simulink model "final_quadruped_120722"  (R2021a)
settings: Solver=ode15s  StartTime=0.0  StopTime=10  FixedStep=1e-3  RelTol=1e-5  EnableMultiTasking=on
values from neighbouring files (symbols this model uses):
  foot_x = 8    [bipedparameters.m]    (also in fcn.m; finalrobotParameters.m; finalrobotParameters_110522.m; finalrobotParameters_140522.m)
  foot_y = 6    [bipedparameters.m]    (also in fcn.m; finalrobotParameters.m; finalrobotParameters_110522.m; finalrobotParameters_140522.m)
  foot_z = 1    [bipedparameters.m]    (also in fcn.m; finalrobotParameters.m; finalrobotParameters_110522.m; finalrobotParameters_140522.m)
  height_plane = 0.025    [bipedparameters.m]    (also in finalrobotParameters.m; finalrobotParameters_110522.m; finalrobotParameters_140522.m; finalrobotParameters_240522.m)
  kd_ankle = 1000    [bipedparameters.m]    (also in finalrobotParameters_240522.m)
  kd_hip = 1000    [bipedparameters.m]    (also in finalrobotParameters_240522.m)
  kd_knee = 1000    [bipedparameters.m]    (also in finalrobotParameters_240522.m)
  ki_ankle = 1000    [bipedparameters.m]    (also in finalrobotParameters_240522.m)
  ki_hip = 1000    [bipedparameters.m]    (also in finalrobotParameters_240522.m)
  ki_knee = 2000    [bipedparameters.m]    (also in finalrobotParameters_240522.m)
  kp_ankle = 1000    [bipedparameters.m]    (also in finalrobotParameters_240522.m)
  kp_hip = 1000    [bipedparameters.m]    (also in finalrobotParameters_240522.m)
  kp_knee = 2000    [bipedparameters.m]    (also in finalrobotParameters_240522.m)
  lower_leg_length = 10    [bipedparameters.m]    (also in fcn.m; finalrobotParameters.m; finalrobotParameters_110522.m; finalrobotParameters_140522.m)
  plane_x = 25    [bipedparameters.m]    (also in finalrobotParameters.m; finalrobotParameters_110522.m; finalrobotParameters_140522.m; finalrobotParameters_240522.m)
  plane_y = 3    [bipedparameters.m]    (also in finalrobotParameters.m; finalrobotParameters_110522.m; finalrobotParameters_140522.m; finalrobotParameters_240522.m)
  torso_offset_x = -0.5    [bipedparameters.m]    (also in finalrobotParameters.m = 10; finalrobotParameters_110522.m = 10; finalrobotParameters_140522.m = 10; finalrobotParameters_240522.m = 10)
  torso_offset_z = -2    [bipedparameters.m]    (also in finalrobotParameters.m; finalrobotParameters_110522.m; finalrobotParameters_140522.m; finalrobotParameters_240522.m)
  torso_x = 5    [bipedparameters.m]    (also in fcn.m = 25; finalrobotParameters.m = 25; finalrobotParameters_110522.m = 25; finalrobotParameters_140522.m = 25)
  torso_y = 10    [bipedparameters.m]    (also in fcn.m = 16; finalrobotParameters.m = 16; finalrobotParameters_110522.m = 16; finalrobotParameters_140522.m = 16)
  torso_z = 8    [bipedparameters.m]    (also in fcn.m = 10; finalrobotParameters.m = 10; finalrobotParameters_110522.m = 10; finalrobotParameters_140522.m = 10)
  upper_leg_length = 10    [bipedparameters.m]    (also in fcn.m; finalrobotParameters.m; finalrobotParameters_110522.m; finalrobotParameters_140522.m)
undefined symbols (not defined in the file or in its folder): sigbuilder_block, X, Y, Z
libraries: nesl_utility x288, sm_lib x75, pid_lib x20, Contact_Forces_Lib x16, fl_lib x3
(part 2 of 9)

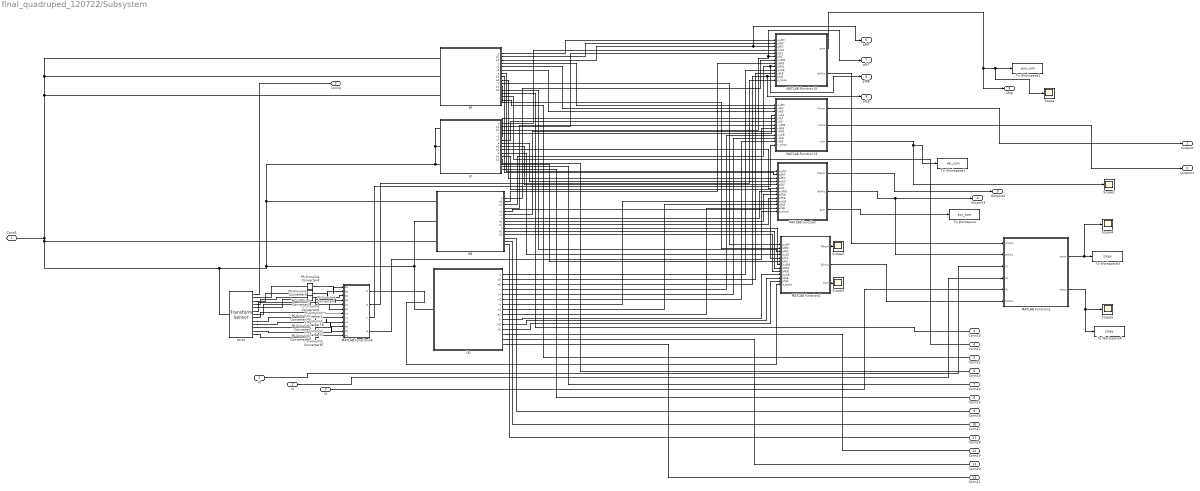
== system final_quadruped_120722/Subsystem ==
  I3 : Inport
  I4 : Inport  Port=2
  I5 : Inport  Port=3
  " RF" : Subsystem
  LB : Subsystem
  LF : Subsystem
  MATLAB Function : MATLAB Function  TreatAsAtomicUnit=on
  MATLAB Function1 : MATLAB Function  TreatAsAtomicUnit=on
  MATLAB Function13 : MATLAB Function  TreatAsAtomicUnit=on
  MATLAB Function14 : MATLAB Function  TreatAsAtomicUnit=on
  MATLAB Function15 : MATLAB Function  TreatAsAtomicUnit=on
  MATLAB Function2 : MATLAB Function  TreatAsAtomicUnit=on
  PS-Simulink Converter{,1..6,76..78,86..87} (12 alike) : nesl_utility/PS-Simulink Converter  PhysicalDomain=network_engine_domain  SubClassName=ps_output  LeftPortType=input  RightPortType=output  PseudoPeriodic=off  Frequencies=[]  Unit=inherit  AffineConversion=off
      settings: SourceProductBaseCode=PW,SS
  RB : Subsystem
  Scope{,1..5} (6 alike) : Scope
  To Workspace : ToWorkspace  VariableName=acc_com  SaveFormat=Timeseries  SampleTime=-1
  To Workspace1 : ToWorkspace  VariableName=vel_com  SaveFormat=Timeseries  SampleTime=-1
  To Workspace2 : ToWorkspace  VariableName=pos_com  SaveFormat=Timeseries  SampleTime=-1
  To Workspace3 : ToWorkspace  VariableName=zmpx  SaveFormat=Timeseries  SampleTime=-1
  To Workspace4 : ToWorkspace  VariableName=zmpy  SaveFormat=Timeseries  SampleTime=-1
  torso : sm_lib/Frames and Transforms/Transform Sensor  MeasurementFrame=World  SenseAngle=off  SenseAxis=off  SenseAngle1=off  SenseAngle2=off  SenseAngle3=off  SenseQ=off  SenseR=off  SenseOmegaX=off  SenseOmegaY=off  SenseOmegaZ=off  SenseOmega1=off  SenseOmega2=off  SenseOmega3=off  SenseQDot=off  SenseRDot=off  SenseAlphaX=on  SenseAlphaY=on  SenseAlphaZ=on  SenseAlpha1=off  SenseAlpha2=off  SenseAlpha3=off  SenseQDDot=off  SenseRDDot=off  SenseX=on  SenseY=on  SenseZ=on  SenseRad=off  SenseAzim=off  SenseDist=off  SenseInc=off  SenseXDot=on  SenseYDot=on  SenseZDot=on  SenseRadDot=off  SenseAzimDot=off  SenseDistDot=off  SenseIncDot=off  SenseXDDot=on  SenseYDDot=on  SenseZDDot=on  SenseRadDDot=off  SenseAzimDDot=off  SenseDistDDot=off  SenseIncDDot=off
  Conn5 : PMIOPort  Side=Left
  Conn4 : PMIOPort  Port=2  Side=Right
  Conn10 : PMIOPort  Port=3  Side=Right
  Conn11 : PMIOPort  Port=4  Side=Right
  Conn12 : PMIOPort  Port=5  Side=Right
  Conn13 : PMIOPort  Port=6  Side=Right
  Conn14 : PMIOPort  Port=7  Side=Right
  Conn15 : PMIOPort  Port=8  Side=Right
  Conn16 : PMIOPort  Port=9  Side=Right
  Conn17 : PMIOPort  Port=10  Side=Right
  Conn18 : PMIOPort  Port=11  Side=Right
  Conn19 : PMIOPort  Port=12  Side=Right
  Conn20 : PMIOPort  Port=13  Side=Right
  Conn21 : PMIOPort  Port=14  Side=Right
  Outport : Outport
  Outport1 : Outport  Port=2
  Outport2 : Outport  Port=3
  Outport3 : Outport  Port=4
  CMg : Outport  Port=5
  pfRF : Outport  Port=6
  pfLF : Outport  Port=7
  pfRB : Outport  Port=8
  pfLB : Outport  Port=9
  wires:
  PS-Simulink Converter3/1 -> MATLAB Function14/4(px)
  PS-Simulink Converter1/1 -> MATLAB Function14/5(py)
  PS-Simulink Converter2/1 -> MATLAB Function14/6(pz)
  MATLAB Function14/3(v) -> MATLAB Function13/13(v_torso)
  MATLAB Function13/1(Mvcm) -> Outport/1
  MATLAB Function13/2(vlinks) -> Outport1/1
  PS-Simulink Converter78/1 -> MATLAB Function14/7(vx)
  PS-Simulink Converter76/1 -> MATLAB Function14/8(vy)
  PS-Simulink Converter77/1 -> MATLAB Function14/9(vz)
  MATLAB Function14/4(a) -> MATLAB Function/13(a_torso)
  MATLAB Function/1(Macm) -> Outport2/1
  MATLAB Function/2(alinks) -> MATLAB Function1/2(alinks), Outport3/1
  MATLAB Function/3(acm) -> To Workspace/1
  MATLAB Function13/3(vcm) -> Scope1/1, To Workspace1/1
  PS-Simulink Converter/1 -> MATLAB Function14/10(ax)
  PS-Simulink Converter87/1 -> MATLAB Function14/11(ay)
  PS-Simulink Converter86/1 -> MATLAB Function14/12(az)
  MATLAB Function14/2(p) -> MATLAB Function15/13(p_torso)
  MATLAB Function15/1(pcm) -> CMg/1, Scope/1, To Workspace2/1
  " RF"/1(p) -> MATLAB Function15/1(pulRF)
  " RF"/2(p1) -> MATLAB Function15/2(pllRF)
  " RF"/3(p2) -> pfRF/1, MATLAB Function15/3(pfRF)
  " RF"/4(v) -> MATLAB Function13/1(vulRF)
  " RF"/5(v1) -> MATLAB Function13/2(vllRF)
  " RF"/6(v2) -> MATLAB Function13/3(vfRF)
  " RF"/7(a) -> MATLAB Function/1(aulRF)
  " RF"/8(a1) -> MATLAB Function/2(allRF)
  " RF"/9(a2) -> MATLAB Function/3(afRF)
  RB/1(p) -> MATLAB Function15/7(pulRB)
  RB/2(p1) -> MATLAB Function15/8(pllRB)
  RB/3(p2) -> pfRB/1, MATLAB Function15/9(pfRB)
  RB/4(v) -> MATLAB Function13/7(vulRB)
  RB/5(v1) -> MATLAB Function13/8(vllRB)
  RB/6(v2) -> MATLAB Function13/9(vfRB)
  RB/7(a) -> MATLAB Function/7(aulRB)
  RB/8(a1) -> MATLAB Function/8(allRB)
  RB/9(a2) -> MATLAB Function/9(afRB)
  LF/1(p) -> MATLAB Function15/4(pulLF)
  LF/2(p1) -> MATLAB Function15/5(pllLF)
  LF/3(p2) -> pfLF/1, MATLAB Function15/6(pfLF)
  LF/4(v) -> MATLAB Function13/4(vulLF)
  LF/5(v1) -> MATLAB Function13/5(vllLF)
  LF/6(v2) -> MATLAB Function13/6(vfLF)
  LF/7(a) -> MATLAB Function/4(aulLF)
  LF/8(a1) -> MATLAB Function/5(allLF)
  LF/9(a2) -> MATLAB Function/6(afLF)
  LB/1(p) -> MATLAB Function15/10(pulLB)
  LB/2(p1) -> MATLAB Function15/11(pllLB)
  LB/3(p2) -> pfLB/1, MATLAB Function15/12(pfLB)
  LB/4(v) -> MATLAB Function13/10(vulLB)
  LB/5(v1) -> MATLAB Function13/11(vllLB)
  LB/6(v2) -> MATLAB Function13/12(vfLB)
  LB/7(a) -> MATLAB Function/10(aulLB)
  LB/8(a1) -> MATLAB Function/11(allLB)
  LB/9(a2) -> MATLAB Function/12(afLB)
  " RF"/10(b) -> MATLAB Function2/1(bulRF)
  " RF"/11(b1) -> MATLAB Function2/2(bllRF)
  " RF"/12(b2) -> MATLAB Function2/3(bfRF)
  LF/10(b) -> MATLAB Function2/4(bulLF)
  LF/11(b1) -> MATLAB Function2/5(bllLF)
  LF/12(b2) -> MATLAB Function2/6(bfLF)
  RB/10(b) -> MATLAB Function2/7(bulRB)
  RB/11(b1) -> MATLAB Function2/8(bllRB)
  RB/12(b2) -> MATLAB Function2/9(bfRB)
  LB/10(b) -> MATLAB Function2/10(bulLB)
  LB/11(b1) -> MATLAB Function2/11(bllLB)
  LB/12(b2) -> MATLAB Function2/12(bfLB)
  PS-Simulink Converter4/1 -> MATLAB Function14/1(bx)
  PS-Simulink Converter5/1 -> MATLAB Function14/2(by)
  PS-Simulink Converter6/1 -> MATLAB Function14/3(bz)
  MATLAB Function14/1(b) -> MATLAB Function2/13(b_torso)
  MATLAB Function15/2(plinks) -> MATLAB Function1/1(plinks)
  MATLAB Function2/2(blinks) -> MATLAB Function1/6(blinks)
  MATLAB Function2/1(Mbcm) -> Scope2/1
  MATLAB Function2/3(bcm) -> Scope3/1
  I3/1 -> MATLAB Function1/3(I3)
  I4/1 -> MATLAB Function1/4(I4)
  I5/1 -> MATLAB Function1/5(I5)
  MATLAB Function1/1(zmpx) -> To Workspace3/1, Scope4/1
  MATLAB Function1/2(zmpy) -> To Workspace4/1, Scope5/1
  connections:
  torso/RConn1 -- Conn4/RConn1
  torso/RConn6 -- PS-Simulink Converter1/LConn1
  torso/RConn5 -- PS-Simulink Converter3/LConn1
  torso/RConn7 -- PS-Simulink Converter2/LConn1
  torso/RConn8 -- PS-Simulink Converter78/LConn1
  torso/RConn9 -- PS-Simulink Converter76/LConn1
  torso/RConn10 -- PS-Simulink Converter77/LConn1
  torso/RConn11 -- PS-Simulink Converter/LConn1
  torso/RConn12 -- PS-Simulink Converter87/LConn1
  torso/RConn13 -- PS-Simulink Converter86/LConn1
  " RF"/RConn1 -- Conn10/RConn1
  Conn11/RConn1 -- " RF"/RConn2
  " RF"/RConn3 -- Conn12/RConn1
  Conn16/RConn1 -- RB/RConn1
  Conn17/RConn1 -- RB/RConn2
  Conn18/RConn1 -- RB/RConn3
  " RF"/LConn3 -- LF/LConn2 -- LF/LConn1 -- LF/LConn3 -- RB/LConn1 -- LB/LConn1 -- RB/LConn2 -- torso/LConn1 -- RB/LConn3 -- Conn5/RConn1 -- " RF"/LConn1 -- " RF"/LConn2
  LF/RConn1 -- Conn13/RConn1
  LF/RConn2 -- Conn14/RConn1
  LF/RConn3 -- Conn15/RConn1
  LB/RConn1 -- Conn19/RConn1
  LB/RConn2 -- Conn20/RConn1
  LB/RConn3 -- Conn21/RConn1
  torso/RConn2 -- PS-Simulink Converter4/LConn1
  torso/RConn3 -- PS-Simulink Converter5/LConn1
  torso/RConn4 -- PS-Simulink Converter6/LConn1

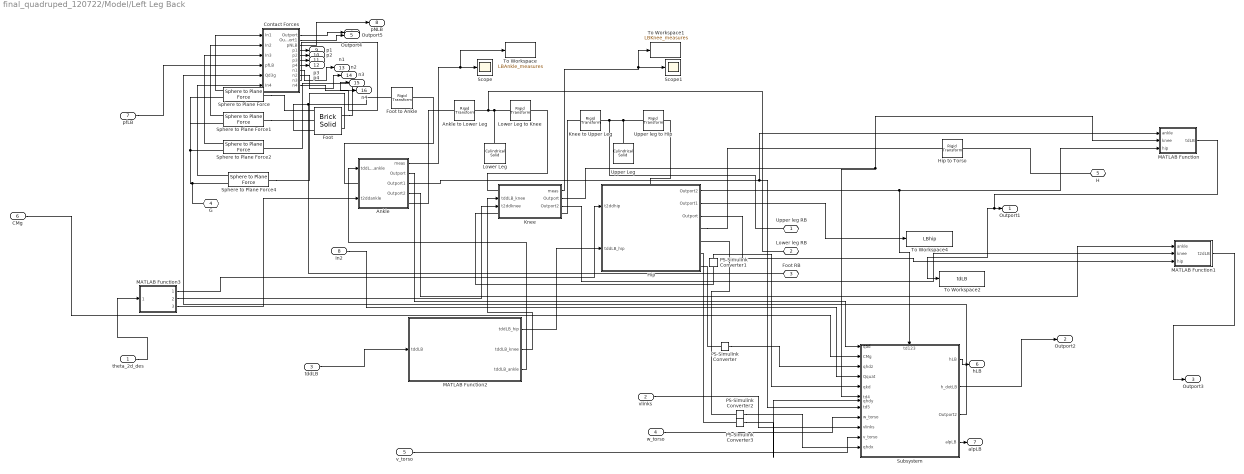
== system final_quadruped_120722/Model/Left Leg Back ==
  theta_2d_des : Inport
  vlinks : Inport  Port=2
  tddLB : Inport  Port=3
  w_torso : Inport  Port=4
  v_torso : Inport  Port=5
  CMg : Inport  Port=6
  pfLB : Inport  Port=7
  In2 : Inport  Port=8
  "Ankle " : Subsystem
      settings: PortSchema="{\"entries\":[{\"content\":{\"sides\":[{\"content\":{\"connectorIds\":[\"In1\",\"LConn1\",\"In2\"]},\"type\":\"ConnectorPlacement.EquallySpacedRectSide\",\"uuid\":\"8820d672-3cef-4e81-999d-8ce69d7112c4\"},{\"content\":{\"connectorIds\":[\"Out1\",\"Out2\",\"Out3\",\"Out4\",\"RConn1\"],\"side\":\"RIGHT\"},\"type\":\"ConnectorPlacement.EquallySpacedRectSide\",\"uuid\":\"2ab010ff-dc37-45a7-8249-0a0b10f28039\"},{\"content\":{\"connectorIds\":[],\"side\":\"TOP\"},\"type\":\"ConnectorPlacement.EquallySpacedRectSide\",\"uuid\":\"2949f9ef-a473-4fca-9f6b-f5ba56dbec95\"}]},\"type\":\"ConnectorPlacement.EquallySpacedConnector\",\"uuid\":\"7b6aa300-a222-434d-a157-d54fa47a17c2\"}],\"packageUris\":[\"http://schema.mathworks.com/mf0/Connector/R2020b\"],\"version\":\"1.0\"}"
  Ankle to Lower Leg : sm_lib/Frames and Transforms/Rigid Transform  TranslationMethod=Cartesian  TranslationStandardOffset=5  TranslationLengthUnit=cm  TranslationStandardAxis=+Y  TranslationCartesianOffset=[0 lower_leg_length/2 0]  TranslationROffset=0  TranslationROffsetUnits=m  TranslationZOffset=0  TranslationZOffsetUnits=m  TranslationThetaOffset=0  TranslationThetaOffsetUnits=deg  RotationMethod=StandardAxis  RotationAngleUnits=deg  RotationStandardAxis=-X  RotationAngle=90  RotationArbitraryAxis=[0 0 1]  FollAlignAxisA=+X  BaseAlignAxisA=+Y  FollAlignAxisB=+Y  BaseAlignAxisB=+Z  RotationSequenceAxes=FollowerAxes  RotationSequence=XYX  RotationSequenceAngles=[0 0 0]  RotationSequenceAnglesUnits=deg  RotationMatrix=[1 0 0; 0 1 0; 0 0 1]
  "Contact Forces " : Subsystem
  Foot : sm_lib/Body Elements/Brick Solid  GraphicAmbientColor=[0.15 0.15 0.15 1.0]  BasedOnType=Density  BrickDimensions=[foot_x foot_y foot_z]  BrickDimensionUnits=cm  CenterOfMass=[0 0 0]  CenterOfMassUnits=m  GraphicDiffuseColor=[0.5 0.5 0.5]  Density=foot_density  DensityUnits=kg/m^3  DoExposeReferenceFrame=off  GraphicEmissiveColor=[0.0 0.0 0.0 1.0]  ExportEntireGeometry=off  SerializedFrames=<Frames><Frame><Id>Frame1</Id><Value><Name>F1</Name><Origin><Source>GeometricFeature</Source><FeatureName>+x -y -z point</FeatureName></Origin><PrimaryAxis><DefinedDirection>+Z</DefinedDirection><Source>ReferenceFrame</Source><SourceDirection>+Z</SourceDirection><FeatureName></FeatureName></PrimaryAxis><SecondaryAxis><DefinedDirection>+X</DefinedDirection><Source>ReferenceFrame</Source><SourceDirection>+X</SourceDirection><FeatureName></FeatureName></SecondaryAxis></Value></Frame><Frame><Id>Frame2</Id><Value><Name>F2</Name><Origin><Source>GeometricFeature</Source><FeatureName>-x -y -z point</FeatureName></Origin><PrimaryAxis><DefinedDirection>+Z</DefinedDirection><Source>ReferenceFrame</Source><SourceDirection>+Z</SourceDirection><FeatureName></FeatureName></PrimaryAxis><SecondaryAxis><DefinedDirection>+X</DefinedDirection><Source>ReferenceFrame</Source><SourceDirection>+X</SourceDirection><FeatureName></FeatureName></SecondaryAxis></Value></Frame><Frame><Id>Frame3</Id><Value><Name>F3</Name><Origin><Source>GeometricFeature</Source><FeatureName>+x +y -z point</FeatureName></Origin><PrimaryAxis><DefinedDirection>+Z</DefinedDirection><Source>ReferenceFrame</Source><SourceDirection>+Z</SourceDirection><FeatureName></FeatureName></PrimaryAxis><SecondaryAxis><DefinedDirection>+X</DefinedDirection><Source>ReferenceFrame</Source><SourceDirection>+X</SourceDirection><FeatureName></FeatureName></SecondaryAxis></Value></Frame><Frame><Id>Frame4</Id><Value><Name>F4</Name><Origin><Source>GeometricFeature</Source><FeatureName>-x +y -z point</FeatureName></Origin><PrimaryAxis><DefinedDirection>+Z</DefinedDirection><Source>ReferenceFrame</Source><SourceDirection>+Z</SourceDirection><FeatureName></FeatureName></PrimaryAxis><SecondaryAxis><DefinedDirection>+X</DefinedDirection><Source>ReferenceFrame</Source><SourceDirection>+X</SourceDirection><FeatureName></FeatureName></SecondaryAxis></Value></Frame><Frame><Id>Frame5</Id><Value><Name>B</Name><Origin><Source>GeometricFeature</Source><FeatureName>+z surface</FeatureName></Origin><PrimaryAxis><DefinedDirection>+Z</DefinedDirection><Source>ReferenceFrame</Source><SourceDirection>-Y</SourceDirection><FeatureName></FeatureName></PrimaryAxis><SecondaryAxis><DefinedDirection>+X</DefinedDirection><Source>ReferenceFrame</Source><SourceDirection>+X</SourceDirection><FeatureName></FeatureName></SecondaryAxis></Value></Frame></Frames>  MarkerShape=Sphere  MarkerSize=10  GraphicType=FromGeometry  InertiaType=CalculateFromGeometry  Mass=1  MassUnits=kg  MomentsOfInertia=[1 1 1]  MomentsOfInertiaUnits=kg*m^2  GraphicOpacity=1.0  ProductsOfInertia=[1 1 1]  ProductsOfInertiaUnits=kg*m^2  GraphicShininess=75  GraphicSpecularColor=[0.5 0.5 0.5 1.0]  GraphicVisPropType=SimpleVisualProperties
  Foot to Ankle : sm_lib/Frames and Transforms/Rigid Transform  TranslationMethod=Cartesian  TranslationStandardOffset=0  TranslationLengthUnit=cm  TranslationStandardAxis=+Z  TranslationCartesianOffset=foot_offset  TranslationROffset=0  TranslationROffsetUnits=m  TranslationZOffset=0  TranslationZOffsetUnits=m  TranslationThetaOffset=0  TranslationThetaOffsetUnits=deg  RotationMethod=None  RotationAngleUnits=deg  RotationStandardAxis=+X  RotationAngle=90  RotationArbitraryAxis=[0 0 1]  FollAlignAxisA=+X  BaseAlignAxisA=+Y  FollAlignAxisB=+Y  BaseAlignAxisB=+Z  RotationSequenceAxes=FollowerAxes  RotationSequence=XYX  RotationSequenceAngles=[0 0 0]  RotationSequenceAnglesUnits=deg  RotationMatrix=[1 0 0; 0 1 0; 0 0 1]
  Hip : Subsystem
      settings: PortSchema="{\"entries\":[{\"content\":{\"sides\":[{\"content\":{\"connectorIds\":[\"In1\",\"In2\"]},\"type\":\"ConnectorPlacement.EquallySpacedRectSide\",\"uuid\":\"3c672348-e331-4589-83a8-aa84cb04ec22\"},{\"content\":{\"connectorIds\":[\"Out1\",\"Out2\",\"Out3\",\"RConn1\",\"RConn2\",\"RConn3\",\"RConn4\"],\"side\":\"RIGHT\"},\"type\":\"ConnectorPlacement.EquallySpacedRectSide\",\"uuid\":\"0cc20eac-f861-4ef7-921b-23889a7eea47\"},{\"content\":{\"connectorIds\":[\"LConn1\"],\"side\":\"TOP\"},\"type\":\"ConnectorPlacement.EquallySpacedRectSide\",\"uuid\":\"90940c46-a35e-4cbd-8c5c-08301adb8b47\"}]},\"type\":\"ConnectorPlacement.EquallySpacedConnector\",\"uuid\":\"ac1266b5-f3f5-41bb-99c9-3c0745f7848a\"}],\"packageUris\":[\"http://schema.mathworks.com/mf0/Connector/R2020b\"],\"version\":\"1.0\"}"
  Hip to Torso : sm_lib/Frames and Transforms/Rigid Transform  TranslationMethod=None  TranslationStandardOffset=0  TranslationLengthUnit=m  TranslationStandardAxis=+Z  TranslationCartesianOffset=[0 0 0]  TranslationROffset=0  TranslationROffsetUnits=m  TranslationZOffset=0  TranslationZOffsetUnits=m  TranslationThetaOffset=0  TranslationThetaOffsetUnits=deg  RotationMethod=StandardAxis  RotationAngleUnits=deg  RotationStandardAxis=+X  RotationAngle=-90  RotationArbitraryAxis=[0 0 1]  FollAlignAxisA=+X  BaseAlignAxisA=+Y  FollAlignAxisB=+Y  BaseAlignAxisB=+Z  RotationSequenceAxes=FollowerAxes  RotationSequence=XYX  RotationSequenceAngles=[0 0 0]  RotationSequenceAnglesUnits=deg  RotationMatrix=[1 0 0; 0 1 0; 0 0 1]
  Knee : Subsystem
      settings: PortSchema="{\"entries\":[{\"content\":{\"sides\":[{\"content\":{\"connectorIds\":[\"LConn1\",\"In1\",\"In2\",\"LConn2\"]},\"type\":\"ConnectorPlacement.EquallySpacedRectSide\",\"uuid\":\"3c672348-e331-4589-83a8-aa84cb04ec22\"},{\"content\":{\"connectorIds\":[\"Out1\",\"Out2\",\"Out3\",\"RConn1\"],\"side\":\"RIGHT\"},\"type\":\"ConnectorPlacement.EquallySpacedRectSide\",\"uuid\":\"0cc20eac-f861-4ef7-921b-23889a7eea47\"},{\"content\":{\"connectorIds\":[],\"side\":\"TOP\"},\"type\":\"ConnectorPlacement.EquallySpacedRectSide\",\"uuid\":\"90940c46-a35e-4cbd-8c5c-08301adb8b47\"}]},\"type\":\"ConnectorPlacement.EquallySpacedConnector\",\"uuid\":\"ac1266b5-f3f5-41bb-99c9-3c0745f7848a\"}],\"packageUris\":[\"http://schema.mathworks.com/mf0/Connector/R2020b\"],\"version\":\"1.0\"}"
  Knee to Upper Leg : sm_lib/Frames and Transforms/Rigid Transform  TranslationMethod=Cartesian  TranslationStandardOffset=5  TranslationLengthUnit=cm  TranslationStandardAxis=+Y  TranslationCartesianOffset=[0 upper_leg_length/2 0]  TranslationROffset=0  TranslationROffsetUnits=m  TranslationZOffset=0  TranslationZOffsetUnits=m  TranslationThetaOffset=0  TranslationThetaOffsetUnits=deg  RotationMethod=StandardAxis  RotationAngleUnits=deg  RotationStandardAxis=+X  RotationAngle=-90  RotationArbitraryAxis=[0 0 1]  FollAlignAxisA=+X  BaseAlignAxisA=+Y  FollAlignAxisB=+Y  BaseAlignAxisB=+Z  RotationSequenceAxes=FollowerAxes  RotationSequence=XYX  RotationSequenceAngles=[0 0 0]  RotationSequenceAnglesUnits=deg  RotationMatrix=[1 0 0; 0 1 0; 0 0 1]
  Lower Leg : sm_lib/Body Elements/Cylindrical Solid  GraphicAmbientColor=[0.15 0.15 0.15 1.0]  BasedOnType=Density  CenterOfMass=[0 0 0]  CenterOfMassUnits=m  GraphicDiffuseColor=[0.5 0.5 0.5]  CylinderLength=lower_leg_length  CylinderLengthUnits=cm  CylinderRadius=leg_radius  CylinderRadiusUnits=cm  Density=density  DensityUnits=kg/m^3  DoExposeReferenceFrame=on  GraphicEmissiveColor=[0.0 0.0 0.0 1.0]  ExportEntireGeometry=off  SerializedFrames=<Frames/>  MarkerShape=Sphere  MarkerSize=10  GraphicType=FromGeometry  InertiaType=CalculateFromGeometry  Mass=1  MassUnits=kg  MomentsOfInertia=[1 1 1]  MomentsOfInertiaUnits=kg*m^2  GraphicOpacity=1.0  ProductsOfInertia=[1 1 1]  ProductsOfInertiaUnits=kg*m^2  GraphicShininess=75  GraphicSpecularColor=[0.5 0.5 0.5 1.0]  GraphicVisPropType=SimpleVisualProperties
  Lower Leg to Knee : sm_lib/Frames and Transforms/Rigid Transform  TranslationMethod=Cartesian  TranslationStandardOffset=5  TranslationLengthUnit=cm  TranslationStandardAxis=+Z  TranslationCartesianOffset=[0 0 lower_leg_length/2]  TranslationROffset=0  TranslationROffsetUnits=m  TranslationZOffset=0  TranslationZOffsetUnits=m  TranslationThetaOffset=0  TranslationThetaOffsetUnits=deg  RotationMethod=StandardAxis  RotationAngleUnits=deg  RotationStandardAxis=+X  RotationAngle=90  RotationArbitraryAxis=[0 0 1]  FollAlignAxisA=+X  BaseAlignAxisA=+Y  FollAlignAxisB=+Y  BaseAlignAxisB=+Z  RotationSequenceAxes=FollowerAxes  RotationSequence=XYX  RotationSequenceAngles=[0 0 0]  RotationSequenceAnglesUnits=deg  RotationMatrix=[1 0 0; 0 1 0; 0 0 1]
  MATLAB Function : MATLAB Function  TreatAsAtomicUnit=on
  MATLAB Function1 : MATLAB Function  TreatAsAtomicUnit=on
  MATLAB Function2 : MATLAB Function  TreatAsAtomicUnit=on
  MATLAB Function3 : MATLAB Function  TreatAsAtomicUnit=on
  PS-Simulink Converter{,1..3} (4 alike) : nesl_utility/PS-Simulink Converter  PhysicalDomain=network_engine_domain  SubClassName=ps_output  LeftPortType=input  RightPortType=output  PseudoPeriodic=off  Frequencies=[]  Unit=inherit  AffineConversion=off
      settings: SourceProductBaseCode=PW,SS
  Scope : Scope
  Scope1 : Scope
  Sphere to Plane Force : Contact_Forces_Lib/3D/Sphere to Plane Force  sphere_rad=contact_point_radius  plane_lenx=plane_x  plane_leny=plane_y  plane_depth=height_plane/2  force_law=Linear  k_contact=contact_stiffness  b_contact=contact_damping  pen_full_damp_F=1e-4  pen_exponent=1  custom_param_1=1  custom_param_2=1  friction_law=Stick-Slip Continuous  mu_kinetic=mu_k  mu_static=mu_s  v_thr=mu_vth  vis_on=on  vis_opc_en=0  vis_len_plaBz=0.005  vis_clr=[0.9 0.2 0.2]  vis_opc=0.7
  Sphere to Plane Force1 : Contact_Forces_Lib/3D/Sphere to Plane Force  sphere_rad=contact_point_radius  plane_lenx=plane_x  plane_leny=plane_y  plane_depth=height_plane/2  force_law=Linear  k_contact=contact_stiffness  b_contact=contact_damping  pen_full_damp_F=1e-4  pen_exponent=1  custom_param_1=1  custom_param_2=1  friction_law=Stick-Slip Continuous  mu_kinetic=mu_k  mu_static=mu_s  v_thr=mu_vth  vis_on=off  vis_opc_en=0  vis_len_plaBz=0.005  vis_clr=[0.9 0.2 0.2]  vis_opc=0.7
  Sphere to Plane Force2 : Contact_Forces_Lib/3D/Sphere to Plane Force  sphere_rad=contact_point_radius  plane_lenx=plane_x  plane_leny=plane_y  plane_depth=height_plane/2  force_law=Linear  k_contact=contact_stiffness  b_contact=contact_damping  pen_full_damp_F=1e-4  pen_exponent=1  custom_param_1=1  custom_param_2=1  friction_law=Stick-Slip Continuous  mu_kinetic=mu_k  mu_static=mu_s  v_thr=mu_vth  vis_on=off  vis_opc_en=0  vis_len_plaBz=0.005  vis_clr=[0.9 0.2 0.2]  vis_opc=0.7
  Sphere to Plane Force4 : Contact_Forces_Lib/3D/Sphere to Plane Force  sphere_rad=contact_point_radius  plane_lenx=plane_x  plane_leny=plane_y  plane_depth=height_plane/2  force_law=Linear  k_contact=contact_stiffness  b_contact=contact_damping  pen_full_damp_F=1e-4  pen_exponent=1  custom_param_1=1  custom_param_2=1  friction_law=Stick-Slip Continuous  mu_kinetic=mu_k  mu_static=mu_s  v_thr=mu_vth  vis_on=off  vis_opc_en=0  vis_len_plaBz=0.005  vis_clr=[0.9 0.2 0.2]  vis_opc=0.7
  Subsystem : Subsystem
      settings: PortSchema="{\"entries\":[{\"content\":{\"sides\":[{\"content\":{\"connectorIds\":[\"In1\",\"In2\",\"In3\",\"In4\",\"In5\",\"In6\",\"In7\",\"In8\",\"In9\",\"In10\",\"In11\",\"In12\"]},\"type\":\"ConnectorPlacement.EquallySpacedRectSide\",\"uuid\":\"86ce1042-93a3-4257-9482-b934ed56108e\"},{\"content\":{\"connectorIds\":[\"Out1\",\"Out2\",\"Out3\",\"Out4\"],\"side\":\"RIGHT\"},\"type\":\"ConnectorPlacement.EquallySpacedRectSide\",\"uuid\":\"9186dd22-c036-4814-9c8f-a02c82466cca\"},{\"content\":{\"connectorIds\":[\"In13\"],\"side\":\"TOP\"},\"type\":\"ConnectorPlacement.EquallySpacedRectSide\",\"uuid\":\"8b91f2be-4c09-4acb-8fc1-b217aa758295\"}]},\"type\":\"ConnectorPlacement.EquallySpacedConnector\",\"uuid\":\"b7c3f053-f66c-40d9-bf5a-575a18fb37e5\"}],\"packageUris\":[\"http://schema.mathworks.com/mf0/Connector/R2020b\"],\"version\":\"1.0\"}"
  To Workspace : ToWorkspace  VariableName=LBAnkle_measures  SaveFormat=Timeseries  SampleTime=-1
  To Workspace1 : ToWorkspace  VariableName=LBKnee_measures  SaveFormat=Timeseries  SampleTime=-1
  To Workspace2 : ToWorkspace  VariableName=tdLB  SaveFormat=Timeseries  SampleTime=-1
  To Workspace4 : ToWorkspace  VariableName=LBhip  SaveFormat=Timeseries  SampleTime=-1
  Upper Leg : sm_lib/Body Elements/Cylindrical Solid  GraphicAmbientColor=[0.15 0.15 0.15 1.0]  BasedOnType=Density  CenterOfMass=[0 0 0]  CenterOfMassUnits=m  GraphicDiffuseColor=[0.5 0.5 0.5]  CylinderLength=upper_leg_length  CylinderLengthUnits=cm  CylinderRadius=leg_radius  CylinderRadiusUnits=cm  Density=1000  DensityUnits=kg/m^3  DoExposeReferenceFrame=on  GraphicEmissiveColor=[0.0 0.0 0.0 1.0]  ExportEntireGeometry=off  SerializedFrames=<Frames/>  MarkerShape=Sphere  MarkerSize=10  GraphicType=FromGeometry  InertiaType=CalculateFromGeometry  Mass=1  MassUnits=kg  MomentsOfInertia=[1 1 1]  MomentsOfInertiaUnits=kg*m^2  GraphicOpacity=1.0  ProductsOfInertia=[1 1 1]  ProductsOfInertiaUnits=kg*m^2  GraphicShininess=75  GraphicSpecularColor=[0.5 0.5 0.5 1.0]  GraphicVisPropType=SimpleVisualProperties
  Upper leg to Hip : sm_lib/Frames and Transforms/Rigid Transform  TranslationMethod=Cartesian  TranslationStandardOffset=5  TranslationLengthUnit=cm  TranslationStandardAxis=+Z  TranslationCartesianOffset=[0 0 upper_leg_length/2]  TranslationROffset=0  TranslationROffsetUnits=m  TranslationZOffset=0  TranslationZOffsetUnits=m  TranslationThetaOffset=0  TranslationThetaOffsetUnits=deg  RotationMethod=StandardAxis  RotationAngleUnits=deg  RotationStandardAxis=+X  RotationAngle=90  RotationArbitraryAxis=[0 0 1]  FollAlignAxisA=+X  BaseAlignAxisA=+Y  FollAlignAxisB=+Y  BaseAlignAxisB=+Z  RotationSequenceAxes=FollowerAxes  RotationSequence=XYX  RotationSequenceAngles=[0 0 0]  RotationSequenceAnglesUnits=deg  RotationMatrix=[1 0 0; 0 1 0; 0 0 1]
  Upper leg RB : PMIOPort  Side=Left
  Lower leg RB : PMIOPort  Port=2  Side=Left
  Foot RB : PMIOPort  Port=3  Side=Left
  "G " : PMIOPort  Port=4  Side=Right
  H : PMIOPort  Port=5  Side=Right
  Outport1 : Outport
  Outport2 : Outport  Port=2
  Outport3 : Outport  Port=3
  Outport4 : Outport  Port=4
  Outport5 : Outport  Port=5
  hLB : Outport  Port=6
  alpLB : Outport  Port=7
  pNLB : Outport  Port=8
  p1 : Outport  Port=9
  p2 : Outport  Port=10
  p3 : Outport  Port=11
  p4 : Outport  Port=12
  n1 : Outport  Port=13
  n2 : Outport  Port=14
  n3 : Outport  Port=15
  n4 : Outport  Port=16
  wires:
  Sphere to Plane Force/1 -> "Contact Forces "/1(In1)
  Sphere to Plane Force1/1 -> "Contact Forces "/2(In2)
  Sphere to Plane Force2/1 -> "Contact Forces "/3(In3)
  Sphere to Plane Force4/1 -> "Contact Forces "/6(In4)
  "Ankle "/1(meas) -> To Workspace/1, Scope/1
  tddLB/1 -> MATLAB Function2/1(tddLB)
  MATLAB Function2/3(tddLB_ankle) -> "Ankle "/1(tddLB_ankle)
  Knee/1(meas) -> To Workspace1/1, Scope1/1
  MATLAB Function2/2(tddLB_knee) -> Knee/1(tddLB_knee)
  MATLAB Function2/1(tddLB_hip) -> Hip/2(tddLB_hip)
  "Ankle "/2(Outport) -> Subsystem/1(qad)
  In2/1 -> Subsystem/4(Qquat)
  PS-Simulink Converter1/1 -> Subsystem/5(qkd)
  "Ankle "/3(Outport1) -> Subsystem/7(td5), MATLAB Function/1(ankle)
  Knee/2(Outport) -> MATLAB Function/2(knee), Subsystem/6(td4)
  MATLAB Function/1(tdLB) -> To Workspace2/1, Outport1/1
  w_torso/1 -> Subsystem/8(w_torso)
  v_torso/1 -> Subsystem/10(v_torso)
  vlinks/1 -> Subsystem/9(vlinks)
  Subsystem/2(h_dotLB) -> Outport2/1
  "Ankle "/4(Outport2) -> MATLAB Function1/1(ankle)
  Knee/3(Outport2) -> MATLAB Function1/2(knee)
  Hip/1(Outport2) -> Subsystem/13(td123), MATLAB Function/3(hip)
  MATLAB Function1/1(t2dLB) -> Outport3/1
  "Contact Forces "/1(Outport) -> Outport4/1
  "Contact Forces "/2(Outport1) -> Outport5/1
  theta_2d_des/1 -> MATLAB Function3/1(theta_2d_des)
  MATLAB Function3/3(t2ddankle) -> "Ankle "/2(t2ddankle)
  MATLAB Function3/2(t2ddknee) -> Knee/2(t2ddknee)
  MATLAB Function3/1(t2ddhip) -> Hip/1(t2ddhip)
  Subsystem/3(Outport2) -> "Contact Forces "/5(Qd3g)
  PS-Simulink Converter2/1 -> Subsystem/11(qhdx)
  PS-Simulink Converter3/1 -> Subsystem/12(qhdy)
  PS-Simulink Converter/1 -> Subsystem/3(qhdz)
  Hip/2(Outport1) -> To Workspace4/1
  Hip/3(Outport) -> MATLAB Function1/3(hip)
  CMg/1 -> Subsystem/2(CMg)
  Subsystem/1(hLB) -> hLB/1
  Subsystem/4(alpLB) -> alpLB/1
  pfLB/1 -> "Contact Forces "/4(pfLB)
  "Contact Forces "/3(pNLB) -> pNLB/1
  "Contact Forces "/4(p1) -> p1/1
  "Contact Forces "/5(p2) -> p2/1
  "Contact Forces "/6(p3) -> p3/1
  "Contact Forces "/7(p4) -> p4/1
  "Contact Forces "/8(n1) -> n1/1
  "Contact Forces "/9(n2) -> n2/1
  "Contact Forces "/10(n3) -> n3/1
  "Contact Forces "/11(n4) -> n4/1
  connections:
  H/RConn1 -- Hip to Torso/RConn1
  Lower Leg to Knee/LConn1 -- Lower Leg/RConn1 -- Lower leg RB/RConn1 -- Ankle to Lower Leg/RConn1
  Upper leg to Hip/LConn1 -- Upper Leg/RConn1 -- Upper leg RB/RConn1 -- Knee to Upper Leg/RConn1
  Sphere to Plane Force/LConn1 -- Foot/LConn1
  Sphere to Plane Force1/LConn1 -- Foot/LConn2
  Sphere to Plane Force4/LConn1 -- Foot/RConn2
  Sphere to Plane Force2/RConn1 -- Sphere to Plane Force/RConn1 -- Sphere to Plane Force1/RConn1 -- "G "/RConn1 -- Sphere to Plane Force4/RConn1
  "Ankle "/LConn1 -- Foot to Ankle/RConn1
  Ankle to Lower Leg/LConn1 -- "Ankle "/RConn1
  Foot/RConn1 -- Sphere to Plane Force2/LConn1
  Foot/LConn3 -- Foot to Ankle/LConn1 -- Foot RB/RConn1
  Knee/LConn1 -- Lower Leg to Knee/RConn1
  Knee to Upper Leg/LConn1 -- Knee/RConn1
  PS-Simulink Converter1/LConn1 -- Knee/LConn2
  Hip/LConn1 -- Upper leg to Hip/RConn1
  Hip/RConn1 -- Hip to Torso/LConn1
  PS-Simulink Converter2/LConn1 -- Hip/RConn2
  PS-Simulink Converter3/LConn1 -- Hip/RConn3
  PS-Simulink Converter/LConn1 -- Hip/RConn4
